simulink model "problem1_sim"  (R2019a)
settings: Solver=FixedStepAuto  StartTime=4  StopTime=30  FixedStep=1e-3  RelTol=1e-3
values from neighbouring files (symbols this model uses):
  beta = .8    (= 0.8)    [problem_1.m]
  k = 7    [problem_1.m]    (also in problem_3.m = B'*s_inf)
  x_0 = 5    [problem_1.m]
settings Model: Creator=glitch  LastModifiedBy=glitch
settings SolverCC: ZeroCrossAlgorithm=Adaptive
settings DebuggingCC: IgnoredZcDiagnostic=none

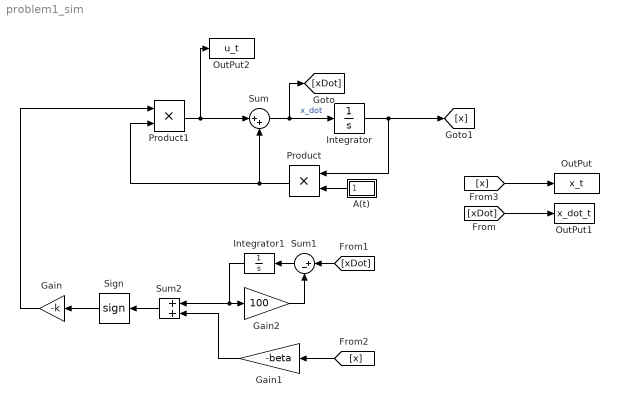
== system problem1_sim ==
  A(t) : Subsystem
  Gain : Gain  Gain=-k
  Gain1 : Gain  Gain=-beta
  Gain2 : Gain  Gain=100
  Integrator : Integrator  InitialCondition=x_0
  Integrator1 : Integrator  InitialCondition=x_0
  OutPut : ToWorkspace  VariableName=x_t  SaveFormat=Structure With Time  SampleTime=-1
  OutPut1 : ToWorkspace  VariableName=x_dot_t  SaveFormat=Structure With Time  SampleTime=-1
  OutPut2 : ToWorkspace  VariableName=u_t  SaveFormat=Structure With Time  SampleTime=-1
  Product : Product
  Product1 : Product
  Sign : Signum
  Sum : Sum  Inputs=|++
  Sum1 : Sum  Inputs=|+-
  Sum2 : Sum
  wires:
  Integrator/1 -> Product/1, [x]
  Product/1 -> Product1/2, Sum/2
  Sum/1 -> [xDot], Integrator/1  "x_dot"
  Product1/1 -> OutPut2/1, Sum/1
  Gain/1 -> Product1/1
  Gain1/1 -> Sum2/2
  Sign/1 -> Gain/1
  Sum1/1 -> Integrator1/1
  Integrator1/1 -> Sum2/1, Gain2/1
  Gain2/1 -> Sum1/2
  Sum2/1 -> Sign/1
  [xDot] -> OutPut1/1
  [xDot] -> Sum1/1
  [x] -> Gain1/1
  [x] -> OutPut/1
  A(t)/1(Out1) -> Product/2

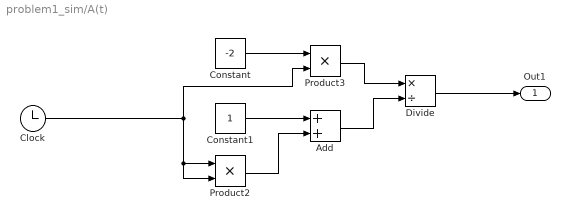
== system problem1_sim/A(t) ==
  Add : Sum
  Clock : Clock
  Constant : Constant  Value=-2
  Constant1 : Constant
  Divide : Product  Inputs=*/
  Product2 : Product
  Product3 : Product
  Out1 : Outport
  wires:
  Constant/1 -> Product3/1
  Constant1/1 -> Add/1
  Clock/1 -> Product3/2, Product2/2, Product2/1
  Product3/1 -> Divide/1
  Add/1 -> Divide/2
  Divide/1 -> Out1/1
  Product2/1 -> Add/2
